simulink model "c00020M_harness"  (R2018a)
settings: Solver=ode3  StartTime=0.0  StopTime=10.0  RelTol=1e-3  EnableMultiTasking=on
undefined symbols (not defined in the file): b, DiscIntNeverNeededParam, J, K, L, PosMinimaW4, R, sigbuilder_block
(part 13 of 41)

== system c00020M_harness/M116/S1 ==
  PhyMeasure : Inport
  SensorOut : Outport
  wires:
  PhyMeasure/1 -> SensorOut/1

== system c00020M_harness/M116/S2 ==
  PhyMeasure : Inport
  SensorOut : Outport
  wires:
  PhyMeasure/1 -> SensorOut/1

== system c00020M_harness/M116/S4 ==
  PhyMeasure : Inport
  SensorOut : Outport
  wires:
  PhyMeasure/1 -> SensorOut/1

== system c00020M_harness/M118/Cyber ==
  note: Sensors
  note: Inputs For Window1
  note: Inputs for Window 2
  note: Inputs for window 3
  note: Inputs for window 4
  note: Users
  note: Users
  note: Sensors
  note: Users
  note: Sensors
  note: Users
  note: Sensors
  note: USERS
      | ---------------------------------
      | 0: None
      | 1: Ventana Arriba
      | 2: Ventana hasta arriba
      | 3: Ventana abajo
      | 4: Ventana hasta abajo
  note: 1: SUBE
      | 0: PARADO
      | -1 BAJA
  note: D = Driver (W1)
      | P1 = Passenger 1 (W2)
      | P2 = Passenger 2 (W3)
      | P3 = Passenger 3 (W4)
      | O = Obstacle
      | C = Control
      | Pri = Prioritizer
      | LD = LockDriver
      | PosW = PositionWindow
      | WL = WindowLogic
      | OW = ObstacleWindow
      | CWXC = ControlWindowXCentralized
      | S = Sensor
      | L = Lock
      | WPos = WindowPosition
      | M = Memory
      | InW = InputWindow
      | WIn = WindowInput
  PosW1 : Inport
  PosW2 : Inport  Port=2
  PosW4 : Inport  Port=3
  DW1 : Inport  Port=4
  DW4 : Inport  Port=5
  P1W2 : Inport  Port=6
  P3W4 : Inport  Port=7
  OW1 : Inport  Port=8
  OW2 : Inport  Port=9
  OW4 : Inport  Port=10
  LD : Inport  Port=11
  Pri4 : Subsystem
  WL : Subsystem
  WL1 : Subsystem
  WL3 : Subsystem
  W1 : Outport
  W2 : Outport  Port=2
  W4 : Outport  Port=3
  wires:
  WL3/1(WindowLogicOutput) -> W4/1
  Pri4/1(User) -> WL3/2(User)
  OW4/1 -> WL3/3(OW)
  PosW4/1 -> WL3/1(WPos)
  P3W4/1 -> Pri4/2(P)
  DW4/1 -> Pri4/1(D)
  WL1/1(WindowLogicOutput) -> W2/1
  OW2/1 -> WL1/3(OW)
  PosW2/1 -> WL1/1(WPos)
  WL/1(WindowLogicOutput) -> W1/1
  OW1/1 -> WL/3(OW)
  PosW1/1 -> WL/1(WPos)
  LD/1 -> WL3/4(L)
  DW1/1 -> WL/2(User)
  P1W2/1 -> WL1/2(User)

== system c00020M_harness/M118/Physical ==
  InW1 : Inport
  InW2 : Inport  Port=2
  InW4 : Inport  Port=3
  W : Subsystem
  W5 : Subsystem
  W7 : Subsystem
  W1 : Outport
  W2 : Outport  Port=2
  W4 : Outport  Port=3
  wires:
  W7/1(WPos) -> W4/1
  W5/1(WPos) -> W2/1
  W/1(WPos) -> W1/1
  InW4/1 -> W7/1(WIn)
  InW2/1 -> W5/1(WIn)
  InW1/1 -> W/1(WIn)

== system c00020M_harness/M118/S1 ==
  PhyMeasure : Inport
  SensorOut : Outport
  wires:
  PhyMeasure/1 -> SensorOut/1

== system c00020M_harness/M118/S2 ==
  PhyMeasure : Inport
  SensorOut : Outport
  wires:
  PhyMeasure/1 -> SensorOut/1

== system c00020M_harness/M118/S4 ==
  PhyMeasure : Inport
  SensorOut : Outport
  wires:
  PhyMeasure/1 -> SensorOut/1

== system c00020M_harness/M119/Cyber ==
  note: Sensors
  note: Inputs For Window1
  note: Inputs for Window 2
  note: Inputs for window 3
  note: Inputs for window 4
  note: Users
  note: Users
  note: Sensors
  note: Users
  note: Sensors
  note: Users
  note: Sensors
  note: USERS
      | ---------------------------------
      | 0: None
      | 1: Ventana Arriba
      | 2: Ventana hasta arriba
      | 3: Ventana abajo
      | 4: Ventana hasta abajo
  note: 1: SUBE
      | 0: PARADO
      | -1 BAJA
  note: D = Driver (W1)
      | P1 = Passenger 1 (W2)
      | P2 = Passenger 2 (W3)
      | P3 = Passenger 3 (W4)
      | O = Obstacle
      | C = Control
      | Pri = Prioritizer
      | LD = LockDriver
      | PosW = PositionWindow
      | WL = WindowLogic
      | OW = ObstacleWindow
      | CWXC = ControlWindowXCentralized
      | S = Sensor
      | L = Lock
      | WPos = WindowPosition
      | M = Memory
      | InW = InputWindow
      | WIn = WindowInput
  PosW1 : Inport
  PosW2 : Inport  Port=2
  PosW4 : Inport  Port=3
  DW1 : Inport  Port=4
  DW4 : Inport  Port=5
  P1W2 : Inport  Port=6
  P3W4 : Inport  Port=7
  OW1 : Inport  Port=8
  OW2 : Inport  Port=9
  OW4 : Inport  Port=10
  LD : Inport  Port=11
  Pri4 : Subsystem
  WL : Subsystem
  WL1 : Subsystem
  WL3 : Subsystem
  W1 : Outport
  W2 : Outport  Port=2
  W4 : Outport  Port=3
  wires:
  WL3/1(WindowLogicOutput) -> W4/1
  Pri4/1(User) -> WL3/2(User)
  OW4/1 -> WL3/3(OW)
  PosW4/1 -> WL3/1(WPos)
  P3W4/1 -> Pri4/2(P)
  DW4/1 -> Pri4/1(D)
  WL1/1(WindowLogicOutput) -> W2/1
  OW2/1 -> WL1/3(OW)
  PosW2/1 -> WL1/1(WPos)
  WL/1(WindowLogicOutput) -> W1/1
  OW1/1 -> WL/3(OW)
  PosW1/1 -> WL/1(WPos)
  LD/1 -> WL3/4(L)
  DW1/1 -> WL/2(User)
  P1W2/1 -> WL1/2(User)

== system c00020M_harness/M119/Physical ==
  InW1 : Inport
  InW2 : Inport  Port=2
  InW4 : Inport  Port=3
  W : Subsystem
  W5 : Subsystem
  W7 : Subsystem
  W1 : Outport
  W2 : Outport  Port=2
  W4 : Outport  Port=3
  wires:
  W7/1(WPos) -> W4/1
  W5/1(WPos) -> W2/1
  W/1(WPos) -> W1/1
  InW4/1 -> W7/1(WIn)
  InW2/1 -> W5/1(WIn)
  InW1/1 -> W/1(WIn)

== system c00020M_harness/M119/S1 ==
  PhyMeasure : Inport
  SensorOut : Outport
  wires:
  PhyMeasure/1 -> SensorOut/1

== system c00020M_harness/M119/S2 ==
  PhyMeasure : Inport
  SensorOut : Outport
  wires:
  PhyMeasure/1 -> SensorOut/1

== system c00020M_harness/M119/S4 ==
  PhyMeasure : Inport
  SensorOut : Outport
  wires:
  PhyMeasure/1 -> SensorOut/1

== system c00020M_harness/M120/Cyber ==
  note: Sensors
  note: Inputs For Window1
  note: Inputs for Window 2
  note: Inputs for window 3
  note: Inputs for window 4
  note: Users
  note: Users
  note: Sensors
  note: Users
  note: Sensors
  note: Users
  note: Sensors
  note: USERS
      | ---------------------------------
      | 0: None
      | 1: Ventana Arriba
      | 2: Ventana hasta arriba
      | 3: Ventana abajo
      | 4: Ventana hasta abajo
  note: 1: SUBE
      | 0: PARADO
      | -1 BAJA
  note: D = Driver (W1)
      | P1 = Passenger 1 (W2)
      | P2 = Passenger 2 (W3)
      | P3 = Passenger 3 (W4)
      | O = Obstacle
      | C = Control
      | Pri = Prioritizer
      | LD = LockDriver
      | PosW = PositionWindow
      | WL = WindowLogic
      | OW = ObstacleWindow
      | CWXC = ControlWindowXCentralized
      | S = Sensor
      | L = Lock
      | WPos = WindowPosition
      | M = Memory
      | InW = InputWindow
      | WIn = WindowInput
  PosW1 : Inport
  PosW2 : Inport  Port=2
  PosW4 : Inport  Port=3
  DW1 : Inport  Port=4
  DW4 : Inport  Port=5
  P1W2 : Inport  Port=6
  P3W4 : Inport  Port=7
  OW1 : Inport  Port=8
  OW2 : Inport  Port=9
  OW4 : Inport  Port=10
  LD : Inport  Port=11
  Pri4 : Subsystem
  WL : Subsystem
  WL1 : Subsystem
  WL3 : Subsystem
  W1 : Outport
  W2 : Outport  Port=2
  W4 : Outport  Port=3
  wires:
  WL3/1(WindowLogicOutput) -> W4/1
  Pri4/1(User) -> WL3/2(User)
  OW4/1 -> WL3/3(OW)
  PosW4/1 -> WL3/1(WPos)
  P3W4/1 -> Pri4/2(P)
  DW4/1 -> Pri4/1(D)
  WL1/1(WindowLogicOutput) -> W2/1
  OW2/1 -> WL1/3(OW)
  PosW2/1 -> WL1/1(WPos)
  WL/1(WindowLogicOutput) -> W1/1
  OW1/1 -> WL/3(OW)
  PosW1/1 -> WL/1(WPos)
  LD/1 -> WL3/4(L)
  DW1/1 -> WL/2(User)
  P1W2/1 -> WL1/2(User)

== system c00020M_harness/M120/Physical ==
  InW1 : Inport
  InW2 : Inport  Port=2
  InW4 : Inport  Port=3
  W : Subsystem
  W5 : Subsystem
  W7 : Subsystem
  W1 : Outport
  W2 : Outport  Port=2
  W4 : Outport  Port=3
  wires:
  W7/1(WPos) -> W4/1
  W5/1(WPos) -> W2/1
  W/1(WPos) -> W1/1
  InW4/1 -> W7/1(WIn)
  InW2/1 -> W5/1(WIn)
  InW1/1 -> W/1(WIn)

== system c00020M_harness/M120/S1 ==
  PhyMeasure : Inport
  SensorOut : Outport
  wires:
  PhyMeasure/1 -> SensorOut/1

== system c00020M_harness/M120/S2 ==
  PhyMeasure : Inport
  SensorOut : Outport
  wires:
  PhyMeasure/1 -> SensorOut/1

== system c00020M_harness/M120/S4 ==
  PhyMeasure : Inport
  SensorOut : Outport
  wires:
  PhyMeasure/1 -> SensorOut/1

== system c00020M_harness/M122/Cyber ==
  note: Sensors
  note: Inputs For Window1
  note: Inputs for Window 2
  note: Inputs for window 3
  note: Inputs for window 4
  note: Users
  note: Users
  note: Sensors
  note: Users
  note: Sensors
  note: Users
  note: Sensors
  note: USERS
      | ---------------------------------
      | 0: None
      | 1: Ventana Arriba
      | 2: Ventana hasta arriba
      | 3: Ventana abajo
      | 4: Ventana hasta abajo
  note: 1: SUBE
      | 0: PARADO
      | -1 BAJA
  note: D = Driver (W1)
      | P1 = Passenger 1 (W2)
      | P2 = Passenger 2 (W3)
      | P3 = Passenger 3 (W4)
      | O = Obstacle
      | C = Control
      | Pri = Prioritizer
      | LD = LockDriver
      | PosW = PositionWindow
      | WL = WindowLogic
      | OW = ObstacleWindow
      | CWXC = ControlWindowXCentralized
      | S = Sensor
      | L = Lock
      | WPos = WindowPosition
      | M = Memory
      | InW = InputWindow
      | WIn = WindowInput
  PosW1 : Inport
  PosW2 : Inport  Port=2
  PosW4 : Inport  Port=3
  DW1 : Inport  Port=4
  DW4 : Inport  Port=5
  P1W2 : Inport  Port=6
  P3W4 : Inport  Port=7
  OW1 : Inport  Port=8
  OW2 : Inport  Port=9
  OW4 : Inport  Port=10
  LD : Inport  Port=11
  Pri4 : Subsystem
  WL : Subsystem
  WL1 : Subsystem
  WL3 : Subsystem
  W1 : Outport
  W2 : Outport  Port=2
  W4 : Outport  Port=3
  wires:
  WL3/1(WindowLogicOutput) -> W4/1
  Pri4/1(User) -> WL3/2(User)
  OW4/1 -> WL3/3(OW)
  PosW4/1 -> WL3/1(WPos)
  P3W4/1 -> Pri4/2(P)
  DW4/1 -> Pri4/1(D)
  WL1/1(WindowLogicOutput) -> W2/1
  OW2/1 -> WL1/3(OW)
  PosW2/1 -> WL1/1(WPos)
  WL/1(WindowLogicOutput) -> W1/1
  OW1/1 -> WL/3(OW)
  PosW1/1 -> WL/1(WPos)
  LD/1 -> WL3/4(L)
  DW1/1 -> WL/2(User)
  P1W2/1 -> WL1/2(User)

== system c00020M_harness/M122/Physical ==
  InW1 : Inport
  InW2 : Inport  Port=2
  InW4 : Inport  Port=3
  W : Subsystem
  W5 : Subsystem
  W7 : Subsystem
  W1 : Outport
  W2 : Outport  Port=2
  W4 : Outport  Port=3
  wires:
  W7/1(WPos) -> W4/1
  W5/1(WPos) -> W2/1
  W/1(WPos) -> W1/1
  InW4/1 -> W7/1(WIn)
  InW2/1 -> W5/1(WIn)
  InW1/1 -> W/1(WIn)

== system c00020M_harness/M122/S1 ==
  PhyMeasure : Inport
  SensorOut : Outport
  wires:
  PhyMeasure/1 -> SensorOut/1

== system c00020M_harness/M122/S2 ==
  PhyMeasure : Inport
  SensorOut : Outport
  wires:
  PhyMeasure/1 -> SensorOut/1

== system c00020M_harness/M122/S4 ==
  PhyMeasure : Inport
  SensorOut : Outport
  wires:
  PhyMeasure/1 -> SensorOut/1

== system c00020M_harness/M123/Cyber ==
  note: Sensors
  note: Inputs For Window1
  note: Inputs for Window 2
  note: Inputs for window 3
  note: Inputs for window 4
  note: Users
  note: Users
  note: Sensors
  note: Users
  note: Sensors
  note: Users
  note: Sensors
  note: USERS
      | ---------------------------------
      | 0: None
      | 1: Ventana Arriba
      | 2: Ventana hasta arriba
      | 3: Ventana abajo
      | 4: Ventana hasta abajo
  note: 1: SUBE
      | 0: PARADO
      | -1 BAJA
  note: D = Driver (W1)
      | P1 = Passenger 1 (W2)
      | P2 = Passenger 2 (W3)
      | P3 = Passenger 3 (W4)
      | O = Obstacle
      | C = Control
      | Pri = Prioritizer
      | LD = LockDriver
      | PosW = PositionWindow
      | WL = WindowLogic
      | OW = ObstacleWindow
      | CWXC = ControlWindowXCentralized
      | S = Sensor
      | L = Lock
      | WPos = WindowPosition
      | M = Memory
      | InW = InputWindow
      | WIn = WindowInput
  PosW1 : Inport
  PosW2 : Inport  Port=2
  PosW4 : Inport  Port=3
  DW1 : Inport  Port=4
  DW4 : Inport  Port=5
  P1W2 : Inport  Port=6
  P3W4 : Inport  Port=7
  OW1 : Inport  Port=8
  OW2 : Inport  Port=9
  OW4 : Inport  Port=10
  LD : Inport  Port=11
  Pri4 : Subsystem
  WL : Subsystem
  WL1 : Subsystem
  WL3 : Subsystem
  W1 : Outport
  W2 : Outport  Port=2
  W4 : Outport  Port=3
  wires:
  WL3/1(WindowLogicOutput) -> W4/1
  Pri4/1(User) -> WL3/2(User)
  OW4/1 -> WL3/3(OW)
  PosW4/1 -> WL3/1(WPos)
  P3W4/1 -> Pri4/2(P)
  DW4/1 -> Pri4/1(D)
  WL1/1(WindowLogicOutput) -> W2/1
  OW2/1 -> WL1/3(OW)
  PosW2/1 -> WL1/1(WPos)
  WL/1(WindowLogicOutput) -> W1/1
  OW1/1 -> WL/3(OW)
  PosW1/1 -> WL/1(WPos)
  LD/1 -> WL3/4(L)
  DW1/1 -> WL/2(User)
  P1W2/1 -> WL1/2(User)

== system c00020M_harness/M123/Physical ==
  InW1 : Inport
  InW2 : Inport  Port=2
  InW4 : Inport  Port=3
  W : Subsystem
  W5 : Subsystem
  W7 : Subsystem
  W1 : Outport
  W2 : Outport  Port=2
  W4 : Outport  Port=3
  wires:
  W7/1(WPos) -> W4/1
  W5/1(WPos) -> W2/1
  W/1(WPos) -> W1/1
  InW4/1 -> W7/1(WIn)
  InW2/1 -> W5/1(WIn)
  InW1/1 -> W/1(WIn)

== system c00020M_harness/M123/S1 ==
  PhyMeasure : Inport
  SensorOut : Outport
  wires:
  PhyMeasure/1 -> SensorOut/1

== system c00020M_harness/M123/S2 ==
  PhyMeasure : Inport
  SensorOut : Outport
  wires:
  PhyMeasure/1 -> SensorOut/1

== system c00020M_harness/M123/S4 ==
  PhyMeasure : Inport
  SensorOut : Outport
  wires:
  PhyMeasure/1 -> SensorOut/1

== system c00020M_harness/M124/Cyber ==
  note: Sensors
  note: Inputs For Window1
  note: Inputs for Window 2
  note: Inputs for window 3
  note: Inputs for window 4
  note: Users
  note: Users
  note: Sensors
  note: Users
  note: Sensors
  note: Users
  note: Sensors
  note: USERS
      | ---------------------------------
      | 0: None
      | 1: Ventana Arriba
      | 2: Ventana hasta arriba
      | 3: Ventana abajo
      | 4: Ventana hasta abajo
  note: 1: SUBE
      | 0: PARADO
      | -1 BAJA
  note: D = Driver (W1)
      | P1 = Passenger 1 (W2)
      | P2 = Passenger 2 (W3)
      | P3 = Passenger 3 (W4)
      | O = Obstacle
      | C = Control
      | Pri = Prioritizer
      | LD = LockDriver
      | PosW = PositionWindow
      | WL = WindowLogic
      | OW = ObstacleWindow
      | CWXC = ControlWindowXCentralized
      | S = Sensor
      | L = Lock
      | WPos = WindowPosition
      | M = Memory
      | InW = InputWindow
      | WIn = WindowInput
  PosW1 : Inport
  PosW2 : Inport  Port=2
  PosW4 : Inport  Port=3
  DW1 : Inport  Port=4
  DW4 : Inport  Port=5
  P1W2 : Inport  Port=6
  P3W4 : Inport  Port=7
  OW1 : Inport  Port=8
  OW2 : Inport  Port=9
  OW4 : Inport  Port=10
  LD : Inport  Port=11
  Pri4 : Subsystem
  WL : Subsystem
  WL1 : Subsystem
  WL3 : Subsystem
  W1 : Outport
  W2 : Outport  Port=2
  W4 : Outport  Port=3
  wires:
  WL3/1(WindowLogicOutput) -> W4/1
  Pri4/1(User) -> WL3/2(User)
  OW4/1 -> WL3/3(OW)
  PosW4/1 -> WL3/1(WPos)
  P3W4/1 -> Pri4/2(P)
  DW4/1 -> Pri4/1(D)
  WL1/1(WindowLogicOutput) -> W2/1
  OW2/1 -> WL1/3(OW)
  PosW2/1 -> WL1/1(WPos)
  WL/1(WindowLogicOutput) -> W1/1
  OW1/1 -> WL/3(OW)
  PosW1/1 -> WL/1(WPos)
  LD/1 -> WL3/4(L)
  DW1/1 -> WL/2(User)
  P1W2/1 -> WL1/2(User)

== system c00020M_harness/M124/Physical ==
  InW1 : Inport
  InW2 : Inport  Port=2
  InW4 : Inport  Port=3
  W : Subsystem
  W5 : Subsystem
  W7 : Subsystem
  W1 : Outport
  W2 : Outport  Port=2
  W4 : Outport  Port=3
  wires:
  W7/1(WPos) -> W4/1
  W5/1(WPos) -> W2/1
  W/1(WPos) -> W1/1
  InW4/1 -> W7/1(WIn)
  InW2/1 -> W5/1(WIn)
  InW1/1 -> W/1(WIn)

== system c00020M_harness/M124/S1 ==
  PhyMeasure : Inport
  SensorOut : Outport
  wires:
  PhyMeasure/1 -> SensorOut/1

== system c00020M_harness/M124/S2 ==
  PhyMeasure : Inport
  SensorOut : Outport
  wires:
  PhyMeasure/1 -> SensorOut/1

== system c00020M_harness/M124/S4 ==
  PhyMeasure : Inport
  SensorOut : Outport
  wires:
  PhyMeasure/1 -> SensorOut/1

== system c00020M_harness/M126/Cyber ==
  note: Sensors
  note: Inputs For Window1
  note: Inputs for Window 2
  note: Inputs for window 3
  note: Inputs for window 4
  note: Users
  note: Users
  note: Sensors
  note: Users
  note: Sensors
  note: Users
  note: Sensors
  note: USERS
      | ---------------------------------
      | 0: None
      | 1: Ventana Arriba
      | 2: Ventana hasta arriba
      | 3: Ventana abajo
      | 4: Ventana hasta abajo
  note: 1: SUBE
      | 0: PARADO
      | -1 BAJA
  note: D = Driver (W1)
      | P1 = Passenger 1 (W2)
      | P2 = Passenger 2 (W3)
      | P3 = Passenger 3 (W4)
      | O = Obstacle
      | C = Control
      | Pri = Prioritizer
      | LD = LockDriver
      | PosW = PositionWindow
      | WL = WindowLogic
      | OW = ObstacleWindow
      | CWXC = ControlWindowXCentralized
      | S = Sensor
      | L = Lock
      | WPos = WindowPosition
      | M = Memory
      | InW = InputWindow
      | WIn = WindowInput
  PosW1 : Inport
  PosW2 : Inport  Port=2
  PosW4 : Inport  Port=3
  DW1 : Inport  Port=4
  DW4 : Inport  Port=5
  P1W2 : Inport  Port=6
  P3W4 : Inport  Port=7
  OW1 : Inport  Port=8
  OW2 : Inport  Port=9
  OW4 : Inport  Port=10
  LD : Inport  Port=11
  Pri4 : Subsystem
  WL : Subsystem
  WL1 : Subsystem
  WL3 : Subsystem
  W1 : Outport
  W2 : Outport  Port=2
  W4 : Outport  Port=3
  wires:
  WL3/1(WindowLogicOutput) -> W4/1
  Pri4/1(User) -> WL3/2(User)
  OW4/1 -> WL3/3(OW)
  PosW4/1 -> WL3/1(WPos)
  P3W4/1 -> Pri4/2(P)
  DW4/1 -> Pri4/1(D)
  WL1/1(WindowLogicOutput) -> W2/1
  OW2/1 -> WL1/3(OW)
  PosW2/1 -> WL1/1(WPos)
  WL/1(WindowLogicOutput) -> W1/1
  OW1/1 -> WL/3(OW)
  PosW1/1 -> WL/1(WPos)
  LD/1 -> WL3/4(L)
  DW1/1 -> WL/2(User)
  P1W2/1 -> WL1/2(User)

== system c00020M_harness/M126/Physical ==
  InW1 : Inport
  InW2 : Inport  Port=2
  InW4 : Inport  Port=3
  W : Subsystem
  W5 : Subsystem
  W7 : Subsystem
  W1 : Outport
  W2 : Outport  Port=2
  W4 : Outport  Port=3
  wires:
  W7/1(WPos) -> W4/1
  W5/1(WPos) -> W2/1
  W/1(WPos) -> W1/1
  InW4/1 -> W7/1(WIn)
  InW2/1 -> W5/1(WIn)
  InW1/1 -> W/1(WIn)

== system c00020M_harness/M126/S1 ==
  PhyMeasure : Inport
  SensorOut : Outport
  wires:
  PhyMeasure/1 -> SensorOut/1

== system c00020M_harness/M126/S2 ==
  PhyMeasure : Inport
  SensorOut : Outport
  wires:
  PhyMeasure/1 -> SensorOut/1

== system c00020M_harness/M126/S4 ==
  PhyMeasure : Inport
  SensorOut : Outport
  wires:
  PhyMeasure/1 -> SensorOut/1

== system c00020M_harness/M127/Cyber ==
  note: Sensors
  note: Inputs For Window1
  note: Inputs for Window 2
  note: Inputs for window 3
  note: Inputs for window 4
  note: Users
  note: Users
  note: Sensors
  note: Users
  note: Sensors
  note: Users
  note: Sensors
  note: USERS
      | ---------------------------------
      | 0: None
      | 1: Ventana Arriba
      | 2: Ventana hasta arriba
      | 3: Ventana abajo
      | 4: Ventana hasta abajo
  note: 1: SUBE
      | 0: PARADO
      | -1 BAJA
  note: D = Driver (W1)
      | P1 = Passenger 1 (W2)
      | P2 = Passenger 2 (W3)
      | P3 = Passenger 3 (W4)
      | O = Obstacle
      | C = Control
      | Pri = Prioritizer
      | LD = LockDriver
      | PosW = PositionWindow
      | WL = WindowLogic
      | OW = ObstacleWindow
      | CWXC = ControlWindowXCentralized
      | S = Sensor
      | L = Lock
      | WPos = WindowPosition
      | M = Memory
      | InW = InputWindow
      | WIn = WindowInput
  PosW1 : Inport
  PosW2 : Inport  Port=2
  PosW4 : Inport  Port=3
  DW1 : Inport  Port=4
  DW4 : Inport  Port=5
  P1W2 : Inport  Port=6
  P3W4 : Inport  Port=7
  OW1 : Inport  Port=8
  OW2 : Inport  Port=9
  OW4 : Inport  Port=10
  LD : Inport  Port=11
  Pri4 : Subsystem
  WL : Subsystem
  WL1 : Subsystem
  WL3 : Subsystem
  W1 : Outport
  W2 : Outport  Port=2
  W4 : Outport  Port=3
  wires:
  WL3/1(WindowLogicOutput) -> W4/1
  Pri4/1(User) -> WL3/2(User)
  OW4/1 -> WL3/3(OW)
  PosW4/1 -> WL3/1(WPos)
  P3W4/1 -> Pri4/2(P)
  DW4/1 -> Pri4/1(D)
  WL1/1(WindowLogicOutput) -> W2/1
  OW2/1 -> WL1/3(OW)
  PosW2/1 -> WL1/1(WPos)
  WL/1(WindowLogicOutput) -> W1/1
  OW1/1 -> WL/3(OW)
  PosW1/1 -> WL/1(WPos)
  LD/1 -> WL3/4(L)
  DW1/1 -> WL/2(User)
  P1W2/1 -> WL1/2(User)

== system c00020M_harness/M127/Physical ==
  InW1 : Inport
  InW2 : Inport  Port=2
  InW4 : Inport  Port=3
  W : Subsystem
  W5 : Subsystem
  W7 : Subsystem
  W1 : Outport
  W2 : Outport  Port=2
  W4 : Outport  Port=3
  wires:
  W7/1(WPos) -> W4/1
  W5/1(WPos) -> W2/1
  W/1(WPos) -> W1/1
  InW4/1 -> W7/1(WIn)
  InW2/1 -> W5/1(WIn)
  InW1/1 -> W/1(WIn)

== system c00020M_harness/M127/S1 ==
  PhyMeasure : Inport
  SensorOut : Outport
  wires:
  PhyMeasure/1 -> SensorOut/1

== system c00020M_harness/M127/S2 ==
  PhyMeasure : Inport
  SensorOut : Outport
  wires:
  PhyMeasure/1 -> SensorOut/1

== system c00020M_harness/M127/S4 ==
  PhyMeasure : Inport
  SensorOut : Outport
  wires:
  PhyMeasure/1 -> SensorOut/1

== system c00020M_harness/M128/Cyber ==
  note: Sensors
  note: Inputs For Window1
  note: Inputs for Window 2
  note: Inputs for window 3
  note: Inputs for window 4
  note: Users
  note: Users
  note: Sensors
  note: Users
  note: Sensors
  note: Users
  note: Sensors
  note: USERS
      | ---------------------------------
      | 0: None
      | 1: Ventana Arriba
      | 2: Ventana hasta arriba
      | 3: Ventana abajo
      | 4: Ventana hasta abajo
  note: 1: SUBE
      | 0: PARADO
      | -1 BAJA
  note: D = Driver (W1)
      | P1 = Passenger 1 (W2)
      | P2 = Passenger 2 (W3)
      | P3 = Passenger 3 (W4)
      | O = Obstacle
      | C = Control
      | Pri = Prioritizer
      | LD = LockDriver
      | PosW = PositionWindow
      | WL = WindowLogic
      | OW = ObstacleWindow
      | CWXC = ControlWindowXCentralized
      | S = Sensor
      | L = Lock
      | WPos = WindowPosition
      | M = Memory
      | InW = InputWindow
      | WIn = WindowInput
  PosW1 : Inport
  PosW2 : Inport  Port=2
  PosW4 : Inport  Port=3
  DW1 : Inport  Port=4
  DW4 : Inport  Port=5
  P1W2 : Inport  Port=6
  P3W4 : Inport  Port=7
  OW1 : Inport  Port=8
  OW2 : Inport  Port=9
  OW4 : Inport  Port=10
  LD : Inport  Port=11
  Pri4 : Subsystem
  WL : Subsystem
  WL1 : Subsystem
  WL3 : Subsystem
  W1 : Outport
  W2 : Outport  Port=2
  W4 : Outport  Port=3
  wires:
  WL3/1(WindowLogicOutput) -> W4/1
  Pri4/1(User) -> WL3/2(User)
  OW4/1 -> WL3/3(OW)
  PosW4/1 -> WL3/1(WPos)
  P3W4/1 -> Pri4/2(P)
  DW4/1 -> Pri4/1(D)
  WL1/1(WindowLogicOutput) -> W2/1
  OW2/1 -> WL1/3(OW)
  PosW2/1 -> WL1/1(WPos)
  WL/1(WindowLogicOutput) -> W1/1
  OW1/1 -> WL/3(OW)
  PosW1/1 -> WL/1(WPos)
  LD/1 -> WL3/4(L)
  DW1/1 -> WL/2(User)
  P1W2/1 -> WL1/2(User)

== system c00020M_harness/M128/Physical ==
  InW1 : Inport
  InW2 : Inport  Port=2
  InW4 : Inport  Port=3
  W : Subsystem
  W5 : Subsystem
  W7 : Subsystem
  W1 : Outport
  W2 : Outport  Port=2
  W4 : Outport  Port=3
  wires:
  W7/1(WPos) -> W4/1
  W5/1(WPos) -> W2/1
  W/1(WPos) -> W1/1
  InW4/1 -> W7/1(WIn)
  InW2/1 -> W5/1(WIn)
  InW1/1 -> W/1(WIn)

== system c00020M_harness/M128/S1 ==
  PhyMeasure : Inport
  SensorOut : Outport
  wires:
  PhyMeasure/1 -> SensorOut/1

== system c00020M_harness/M128/S2 ==
  PhyMeasure : Inport
  SensorOut : Outport
  wires:
  PhyMeasure/1 -> SensorOut/1

== system c00020M_harness/M128/S4 ==
  PhyMeasure : Inport
  SensorOut : Outport
  wires:
  PhyMeasure/1 -> SensorOut/1

== system c00020M_harness/M130/Cyber ==
  note: Sensors
  note: Inputs For Window1
  note: Inputs for Window 2
  note: Inputs for window 3
  note: Inputs for window 4
  note: Users
  note: Users
  note: Sensors
  note: Users
  note: Sensors
  note: Users
  note: Sensors
  note: USERS
      | ---------------------------------
      | 0: None
      | 1: Ventana Arriba
      | 2: Ventana hasta arriba
      | 3: Ventana abajo
      | 4: Ventana hasta abajo
  note: 1: SUBE
      | 0: PARADO
      | -1 BAJA
  note: D = Driver (W1)
      | P1 = Passenger 1 (W2)
      | P2 = Passenger 2 (W3)
      | P3 = Passenger 3 (W4)
      | O = Obstacle
      | C = Control
      | Pri = Prioritizer
      | LD = LockDriver
      | PosW = PositionWindow
      | WL = WindowLogic
      | OW = ObstacleWindow
      | CWXC = ControlWindowXCentralized
      | S = Sensor
      | L = Lock
      | WPos = WindowPosition
      | M = Memory
      | InW = InputWindow
      | WIn = WindowInput
  PosW1 : Inport
  PosW2 : Inport  Port=2
  PosW4 : Inport  Port=3
  DW1 : Inport  Port=4
  DW4 : Inport  Port=5
  P1W2 : Inport  Port=6
  P3W4 : Inport  Port=7
  OW1 : Inport  Port=8
  OW2 : Inport  Port=9
  OW4 : Inport  Port=10
  LD : Inport  Port=11
  Pri4 : Subsystem
  WL : Subsystem
  WL1 : Subsystem
  WL3 : Subsystem
  W1 : Outport
  W2 : Outport  Port=2
  W4 : Outport  Port=3
  wires:
  WL3/1(WindowLogicOutput) -> W4/1
  Pri4/1(User) -> WL3/2(User)
  OW4/1 -> WL3/3(OW)
  PosW4/1 -> WL3/1(WPos)
  P3W4/1 -> Pri4/2(P)
  DW4/1 -> Pri4/1(D)
  WL1/1(WindowLogicOutput) -> W2/1
  OW2/1 -> WL1/3(OW)
  PosW2/1 -> WL1/1(WPos)
  WL/1(WindowLogicOutput) -> W1/1
  OW1/1 -> WL/3(OW)
  PosW1/1 -> WL/1(WPos)
  LD/1 -> WL3/4(L)
  DW1/1 -> WL/2(User)
  P1W2/1 -> WL1/2(User)

== system c00020M_harness/M130/Physical ==
  InW1 : Inport
  InW2 : Inport  Port=2
  InW4 : Inport  Port=3
  W : Subsystem
  W5 : Subsystem
  W7 : Subsystem
  W1 : Outport
  W2 : Outport  Port=2
  W4 : Outport  Port=3
  wires:
  W7/1(WPos) -> W4/1
  W5/1(WPos) -> W2/1
  W/1(WPos) -> W1/1
  InW4/1 -> W7/1(WIn)
  InW2/1 -> W5/1(WIn)
  InW1/1 -> W/1(WIn)

== system c00020M_harness/M130/S1 ==
  PhyMeasure : Inport
  SensorOut : Outport
  wires:
  PhyMeasure/1 -> SensorOut/1

== system c00020M_harness/M130/S2 ==
  PhyMeasure : Inport
  SensorOut : Outport
  wires:
  PhyMeasure/1 -> SensorOut/1

== system c00020M_harness/M130/S4 ==
  PhyMeasure : Inport
  SensorOut : Outport
  wires:
  PhyMeasure/1 -> SensorOut/1

== system c00020M_harness/M131/Cyber ==
  note: Sensors
  note: Inputs For Window1
  note: Inputs for Window 2
  note: Inputs for window 3
  note: Inputs for window 4
  note: Users
  note: Users
  note: Sensors
  note: Users
  note: Sensors
  note: Users
  note: Sensors
  note: USERS
      | ---------------------------------
      | 0: None
      | 1: Ventana Arriba
      | 2: Ventana hasta arriba
      | 3: Ventana abajo
      | 4: Ventana hasta abajo
  note: 1: SUBE
      | 0: PARADO
      | -1 BAJA
  note: D = Driver (W1)
      | P1 = Passenger 1 (W2)
      | P2 = Passenger 2 (W3)
      | P3 = Passenger 3 (W4)
      | O = Obstacle
      | C = Control
      | Pri = Prioritizer
      | LD = LockDriver
      | PosW = PositionWindow
      | WL = WindowLogic
      | OW = ObstacleWindow
      | CWXC = ControlWindowXCentralized
      | S = Sensor
      | L = Lock
      | WPos = WindowPosition
      | M = Memory
      | InW = InputWindow
      | WIn = WindowInput
  PosW1 : Inport
  PosW2 : Inport  Port=2
  PosW4 : Inport  Port=3
  DW1 : Inport  Port=4
  DW4 : Inport  Port=5
  P1W2 : Inport  Port=6
  P3W4 : Inport  Port=7
  OW1 : Inport  Port=8
  OW2 : Inport  Port=9
  OW4 : Inport  Port=10
  LD : Inport  Port=11
  Pri4 : Subsystem
  WL : Subsystem
  WL1 : Subsystem
  WL3 : Subsystem
  W1 : Outport
  W2 : Outport  Port=2
  W4 : Outport  Port=3
  wires:
  WL3/1(WindowLogicOutput) -> W4/1
  Pri4/1(User) -> WL3/2(User)
  OW4/1 -> WL3/3(OW)
  PosW4/1 -> WL3/1(WPos)
  P3W4/1 -> Pri4/2(P)
  DW4/1 -> Pri4/1(D)
  WL1/1(WindowLogicOutput) -> W2/1
  OW2/1 -> WL1/3(OW)
  PosW2/1 -> WL1/1(WPos)
  WL/1(WindowLogicOutput) -> W1/1
  OW1/1 -> WL/3(OW)
  PosW1/1 -> WL/1(WPos)
  LD/1 -> WL3/4(L)
  DW1/1 -> WL/2(User)
  P1W2/1 -> WL1/2(User)

== system c00020M_harness/M131/Physical ==
  InW1 : Inport
  InW2 : Inport  Port=2
  InW4 : Inport  Port=3
  W : Subsystem
  W5 : Subsystem
  W7 : Subsystem
  W1 : Outport
  W2 : Outport  Port=2
  W4 : Outport  Port=3
  wires:
  W7/1(WPos) -> W4/1
  W5/1(WPos) -> W2/1
  W/1(WPos) -> W1/1
  InW4/1 -> W7/1(WIn)
  InW2/1 -> W5/1(WIn)
  InW1/1 -> W/1(WIn)

== system c00020M_harness/M131/S1 ==
  PhyMeasure : Inport
  SensorOut : Outport
  wires:
  PhyMeasure/1 -> SensorOut/1

== system c00020M_harness/M131/S2 ==
  PhyMeasure : Inport
  SensorOut : Outport
  wires:
  PhyMeasure/1 -> SensorOut/1

== system c00020M_harness/M131/S4 ==
  PhyMeasure : Inport
  SensorOut : Outport
  wires:
  PhyMeasure/1 -> SensorOut/1

== system c00020M_harness/M132/Cyber ==
  note: Sensors
  note: Inputs For Window1
  note: Inputs for Window 2
  note: Inputs for window 3
  note: Inputs for window 4
  note: Users
  note: Users
  note: Sensors
  note: Users
  note: Sensors
  note: Users
  note: Sensors
  note: USERS
      | ---------------------------------
      | 0: None
      | 1: Ventana Arriba
      | 2: Ventana hasta arriba
      | 3: Ventana abajo
      | 4: Ventana hasta abajo
  note: 1: SUBE
      | 0: PARADO
      | -1 BAJA
  note: D = Driver (W1)
      | P1 = Passenger 1 (W2)
      | P2 = Passenger 2 (W3)
      | P3 = Passenger 3 (W4)
      | O = Obstacle
      | C = Control
      | Pri = Prioritizer
      | LD = LockDriver
      | PosW = PositionWindow
      | WL = WindowLogic
      | OW = ObstacleWindow
      | CWXC = ControlWindowXCentralized
      | S = Sensor
      | L = Lock
      | WPos = WindowPosition
      | M = Memory
      | InW = InputWindow
      | WIn = WindowInput
  PosW1 : Inport
  PosW2 : Inport  Port=2
  PosW4 : Inport  Port=3
  DW1 : Inport  Port=4
  DW4 : Inport  Port=5
  P1W2 : Inport  Port=6
  P3W4 : Inport  Port=7
  OW1 : Inport  Port=8
  OW2 : Inport  Port=9
  OW4 : Inport  Port=10
  LD : Inport  Port=11
  Pri4 : Subsystem
  WL : Subsystem
  WL1 : Subsystem
  WL3 : Subsystem
  W1 : Outport
  W2 : Outport  Port=2
  W4 : Outport  Port=3
  wires:
  WL3/1(WindowLogicOutput) -> W4/1
  Pri4/1(User) -> WL3/2(User)
  OW4/1 -> WL3/3(OW)
  PosW4/1 -> WL3/1(WPos)
  P3W4/1 -> Pri4/2(P)
  DW4/1 -> Pri4/1(D)
  WL1/1(WindowLogicOutput) -> W2/1
  OW2/1 -> WL1/3(OW)
  PosW2/1 -> WL1/1(WPos)
  WL/1(WindowLogicOutput) -> W1/1
  OW1/1 -> WL/3(OW)
  PosW1/1 -> WL/1(WPos)
  LD/1 -> WL3/4(L)
  DW1/1 -> WL/2(User)
  P1W2/1 -> WL1/2(User)

== system c00020M_harness/M132/Physical ==
  InW1 : Inport
  InW2 : Inport  Port=2
  InW4 : Inport  Port=3
  W : Subsystem
  W5 : Subsystem
  W7 : Subsystem
  W1 : Outport
  W2 : Outport  Port=2
  W4 : Outport  Port=3
  wires:
  W7/1(WPos) -> W4/1
  W5/1(WPos) -> W2/1
  W/1(WPos) -> W1/1
  InW4/1 -> W7/1(WIn)
  InW2/1 -> W5/1(WIn)
  InW1/1 -> W/1(WIn)

== system c00020M_harness/M132/S1 ==
  PhyMeasure : Inport
  SensorOut : Outport
  wires:
  PhyMeasure/1 -> SensorOut/1

== system c00020M_harness/M132/S2 ==
  PhyMeasure : Inport
  SensorOut : Outport
  wires:
  PhyMeasure/1 -> SensorOut/1

== system c00020M_harness/M132/S4 ==
  PhyMeasure : Inport
  SensorOut : Outport
  wires:
  PhyMeasure/1 -> SensorOut/1

== system c00020M_harness/M134/Cyber ==
  note: Sensors
  note: Inputs For Window1
  note: Inputs for Window 2
  note: Inputs for window 3
  note: Inputs for window 4
  note: Users
  note: Users
  note: Sensors
  note: Users
  note: Sensors
  note: Users
  note: Sensors
  note: USERS
      | ---------------------------------
      | 0: None
      | 1: Ventana Arriba
      | 2: Ventana hasta arriba
      | 3: Ventana abajo
      | 4: Ventana hasta abajo
  note: 1: SUBE
      | 0: PARADO
      | -1 BAJA
  note: D = Driver (W1)
      | P1 = Passenger 1 (W2)
      | P2 = Passenger 2 (W3)
      | P3 = Passenger 3 (W4)
      | O = Obstacle
      | C = Control
      | Pri = Prioritizer
      | LD = LockDriver
      | PosW = PositionWindow
      | WL = WindowLogic
      | OW = ObstacleWindow
      | CWXC = ControlWindowXCentralized
      | S = Sensor
      | L = Lock
      | WPos = WindowPosition
      | M = Memory
      | InW = InputWindow
      | WIn = WindowInput
  PosW1 : Inport
  PosW2 : Inport  Port=2
  PosW4 : Inport  Port=3
  DW1 : Inport  Port=4
  DW4 : Inport  Port=5
  P1W2 : Inport  Port=6
  P3W4 : Inport  Port=7
  OW1 : Inport  Port=8
  OW2 : Inport  Port=9
  OW4 : Inport  Port=10
  LD : Inport  Port=11
  Pri4 : Subsystem
  WL : Subsystem
  WL1 : Subsystem
  WL3 : Subsystem
  W1 : Outport
  W2 : Outport  Port=2
  W4 : Outport  Port=3
  wires:
  WL3/1(WindowLogicOutput) -> W4/1
  Pri4/1(User) -> WL3/2(User)
  OW4/1 -> WL3/3(OW)
  PosW4/1 -> WL3/1(WPos)
  P3W4/1 -> Pri4/2(P)
  DW4/1 -> Pri4/1(D)
  WL1/1(WindowLogicOutput) -> W2/1
  OW2/1 -> WL1/3(OW)
  PosW2/1 -> WL1/1(WPos)
  WL/1(WindowLogicOutput) -> W1/1
  OW1/1 -> WL/3(OW)
  PosW1/1 -> WL/1(WPos)
  LD/1 -> WL3/4(L)
  DW1/1 -> WL/2(User)
  P1W2/1 -> WL1/2(User)

== system c00020M_harness/M134/Physical ==
  InW1 : Inport
  InW2 : Inport  Port=2
  InW4 : Inport  Port=3
  W : Subsystem
  W5 : Subsystem
  W7 : Subsystem
  W1 : Outport
  W2 : Outport  Port=2
  W4 : Outport  Port=3
  wires:
  W7/1(WPos) -> W4/1
  W5/1(WPos) -> W2/1
  W/1(WPos) -> W1/1
  InW4/1 -> W7/1(WIn)
  InW2/1 -> W5/1(WIn)
  InW1/1 -> W/1(WIn)

== system c00020M_harness/M134/S1 ==
  PhyMeasure : Inport
  SensorOut : Outport
  wires:
  PhyMeasure/1 -> SensorOut/1

== system c00020M_harness/M134/S2 ==
  PhyMeasure : Inport
  SensorOut : Outport
  wires:
  PhyMeasure/1 -> SensorOut/1

== system c00020M_harness/M134/S4 ==
  PhyMeasure : Inport
  SensorOut : Outport
  wires:
  PhyMeasure/1 -> SensorOut/1

== system c00020M_harness/M135/Cyber ==
  note: Sensors
  note: Inputs For Window1
  note: Inputs for Window 2
  note: Inputs for window 3
  note: Inputs for window 4
  note: Users
  note: Users
  note: Sensors
  note: Users
  note: Sensors
  note: Users
  note: Sensors
  note: USERS
      | ---------------------------------
      | 0: None
      | 1: Ventana Arriba
      | 2: Ventana hasta arriba
      | 3: Ventana abajo
      | 4: Ventana hasta abajo
  note: 1: SUBE
      | 0: PARADO
      | -1 BAJA
  note: D = Driver (W1)
      | P1 = Passenger 1 (W2)
      | P2 = Passenger 2 (W3)
      | P3 = Passenger 3 (W4)
      | O = Obstacle
      | C = Control
      | Pri = Prioritizer
      | LD = LockDriver
      | PosW = PositionWindow
      | WL = WindowLogic
      | OW = ObstacleWindow
      | CWXC = ControlWindowXCentralized
      | S = Sensor
      | L = Lock
      | WPos = WindowPosition
      | M = Memory
      | InW = InputWindow
      | WIn = WindowInput
  PosW1 : Inport
  PosW2 : Inport  Port=2
  PosW4 : Inport  Port=3
  DW1 : Inport  Port=4
  DW4 : Inport  Port=5
  P1W2 : Inport  Port=6
  P3W4 : Inport  Port=7
  OW1 : Inport  Port=8
  OW2 : Inport  Port=9
  OW4 : Inport  Port=10
  LD : Inport  Port=11
  Pri4 : Subsystem
  WL : Subsystem
  WL1 : Subsystem
  WL3 : Subsystem
  W1 : Outport
  W2 : Outport  Port=2
  W4 : Outport  Port=3
  wires:
  WL3/1(WindowLogicOutput) -> W4/1
  Pri4/1(User) -> WL3/2(User)
  OW4/1 -> WL3/3(OW)
  PosW4/1 -> WL3/1(WPos)
  P3W4/1 -> Pri4/2(P)
  DW4/1 -> Pri4/1(D)
  WL1/1(WindowLogicOutput) -> W2/1
  OW2/1 -> WL1/3(OW)
  PosW2/1 -> WL1/1(WPos)
  WL/1(WindowLogicOutput) -> W1/1
  OW1/1 -> WL/3(OW)
  PosW1/1 -> WL/1(WPos)
  LD/1 -> WL3/4(L)
  DW1/1 -> WL/2(User)
  P1W2/1 -> WL1/2(User)

== system c00020M_harness/M135/Physical ==
  InW1 : Inport
  InW2 : Inport  Port=2
  InW4 : Inport  Port=3
  W : Subsystem
  W5 : Subsystem
  W7 : Subsystem
  W1 : Outport
  W2 : Outport  Port=2
  W4 : Outport  Port=3
  wires:
  W7/1(WPos) -> W4/1
  W5/1(WPos) -> W2/1
  W/1(WPos) -> W1/1
  InW4/1 -> W7/1(WIn)
  InW2/1 -> W5/1(WIn)
  InW1/1 -> W/1(WIn)

== system c00020M_harness/M135/S1 ==
  PhyMeasure : Inport
  SensorOut : Outport
  wires:
  PhyMeasure/1 -> SensorOut/1

== system c00020M_harness/M135/S2 ==
  PhyMeasure : Inport
  SensorOut : Outport
  wires:
  PhyMeasure/1 -> SensorOut/1

== system c00020M_harness/M135/S4 ==
  PhyMeasure : Inport
  SensorOut : Outport
  wires:
  PhyMeasure/1 -> SensorOut/1

== system c00020M_harness/M136/Cyber ==
  note: Sensors
  note: Inputs For Window1
  note: Inputs for Window 2
  note: Inputs for window 3
  note: Inputs for window 4
  note: Users
  note: Users
  note: Sensors
  note: Users
  note: Sensors
  note: Users
  note: Sensors
  note: USERS
      | ---------------------------------
      | 0: None
      | 1: Ventana Arriba
      | 2: Ventana hasta arriba
      | 3: Ventana abajo
      | 4: Ventana hasta abajo
  note: 1: SUBE
      | 0: PARADO
      | -1 BAJA
  note: D = Driver (W1)
      | P1 = Passenger 1 (W2)
      | P2 = Passenger 2 (W3)
      | P3 = Passenger 3 (W4)
      | O = Obstacle
      | C = Control
      | Pri = Prioritizer
      | LD = LockDriver
      | PosW = PositionWindow
      | WL = WindowLogic
      | OW = ObstacleWindow
      | CWXC = ControlWindowXCentralized
      | S = Sensor
      | L = Lock
      | WPos = WindowPosition
      | M = Memory
      | InW = InputWindow
      | WIn = WindowInput
  PosW1 : Inport
  PosW2 : Inport  Port=2
  PosW4 : Inport  Port=3
  DW1 : Inport  Port=4
  DW4 : Inport  Port=5
  P1W2 : Inport  Port=6
  P3W4 : Inport  Port=7
  OW1 : Inport  Port=8
  OW2 : Inport  Port=9
  OW4 : Inport  Port=10
  LD : Inport  Port=11
  Pri4 : Subsystem
  WL : Subsystem
  WL1 : Subsystem
  WL3 : Subsystem
  W1 : Outport
  W2 : Outport  Port=2
  W4 : Outport  Port=3
  wires:
  WL3/1(WindowLogicOutput) -> W4/1
  Pri4/1(User) -> WL3/2(User)
  OW4/1 -> WL3/3(OW)
  PosW4/1 -> WL3/1(WPos)
  P3W4/1 -> Pri4/2(P)
  DW4/1 -> Pri4/1(D)
  WL1/1(WindowLogicOutput) -> W2/1
  OW2/1 -> WL1/3(OW)
  PosW2/1 -> WL1/1(WPos)
  WL/1(WindowLogicOutput) -> W1/1
  OW1/1 -> WL/3(OW)
  PosW1/1 -> WL/1(WPos)
  LD/1 -> WL3/4(L)
  DW1/1 -> WL/2(User)
  P1W2/1 -> WL1/2(User)

== system c00020M_harness/M136/Physical ==
  InW1 : Inport
  InW2 : Inport  Port=2
  InW4 : Inport  Port=3
  W : Subsystem
  W5 : Subsystem
  W7 : Subsystem
  W1 : Outport
  W2 : Outport  Port=2
  W4 : Outport  Port=3
  wires:
  W7/1(WPos) -> W4/1
  W5/1(WPos) -> W2/1
  W/1(WPos) -> W1/1
  InW4/1 -> W7/1(WIn)
  InW2/1 -> W5/1(WIn)
  InW1/1 -> W/1(WIn)

== system c00020M_harness/M136/S1 ==
  PhyMeasure : Inport
  SensorOut : Outport
  wires:
  PhyMeasure/1 -> SensorOut/1

== system c00020M_harness/M136/S2 ==
  PhyMeasure : Inport
  SensorOut : Outport
  wires:
  PhyMeasure/1 -> SensorOut/1

== system c00020M_harness/M136/S4 ==
  PhyMeasure : Inport
  SensorOut : Outport
  wires:
  PhyMeasure/1 -> SensorOut/1

== system c00020M_harness/M138/Cyber ==
  note: Sensors
  note: Inputs For Window1
  note: Inputs for Window 2
  note: Inputs for window 3
  note: Inputs for window 4
  note: Users
  note: Users
  note: Sensors
  note: Users
  note: Sensors
  note: Users
  note: Sensors
  note: USERS
      | ---------------------------------
      | 0: None
      | 1: Ventana Arriba
      | 2: Ventana hasta arriba
      | 3: Ventana abajo
      | 4: Ventana hasta abajo
  note: 1: SUBE
      | 0: PARADO
      | -1 BAJA
  note: D = Driver (W1)
      | P1 = Passenger 1 (W2)
      | P2 = Passenger 2 (W3)
      | P3 = Passenger 3 (W4)
      | O = Obstacle
      | C = Control
      | Pri = Prioritizer
      | LD = LockDriver
      | PosW = PositionWindow
      | WL = WindowLogic
      | OW = ObstacleWindow
      | CWXC = ControlWindowXCentralized
      | S = Sensor
      | L = Lock
      | WPos = WindowPosition
      | M = Memory
      | InW = InputWindow
      | WIn = WindowInput
  PosW1 : Inport
  PosW2 : Inport  Port=2
  PosW4 : Inport  Port=3
  DW1 : Inport  Port=4
  DW4 : Inport  Port=5
  P1W2 : Inport  Port=6
  P3W4 : Inport  Port=7
  OW1 : Inport  Port=8
  OW2 : Inport  Port=9
  OW4 : Inport  Port=10
  LD : Inport  Port=11
  Pri4 : Subsystem
  WL : Subsystem
  WL1 : Subsystem
  WL3 : Subsystem
  W1 : Outport
  W2 : Outport  Port=2
  W4 : Outport  Port=3
  wires:
  WL3/1(WindowLogicOutput) -> W4/1
  Pri4/1(User) -> WL3/2(User)
  OW4/1 -> WL3/3(OW)
  PosW4/1 -> WL3/1(WPos)
  P3W4/1 -> Pri4/2(P)
  DW4/1 -> Pri4/1(D)
  WL1/1(WindowLogicOutput) -> W2/1
  OW2/1 -> WL1/3(OW)
  PosW2/1 -> WL1/1(WPos)
  WL/1(WindowLogicOutput) -> W1/1
  OW1/1 -> WL/3(OW)
  PosW1/1 -> WL/1(WPos)
  LD/1 -> WL3/4(L)
  DW1/1 -> WL/2(User)
  P1W2/1 -> WL1/2(User)

== system c00020M_harness/M138/Physical ==
  InW1 : Inport
  InW2 : Inport  Port=2
  InW4 : Inport  Port=3
  W : Subsystem
  W5 : Subsystem
  W7 : Subsystem
  W1 : Outport
  W2 : Outport  Port=2
  W4 : Outport  Port=3
  wires:
  W7/1(WPos) -> W4/1
  W5/1(WPos) -> W2/1
  W/1(WPos) -> W1/1
  InW4/1 -> W7/1(WIn)
  InW2/1 -> W5/1(WIn)
  InW1/1 -> W/1(WIn)

== system c00020M_harness/M138/S1 ==
  PhyMeasure : Inport
  SensorOut : Outport
  wires:
  PhyMeasure/1 -> SensorOut/1

== system c00020M_harness/M138/S2 ==
  PhyMeasure : Inport
  SensorOut : Outport
  wires:
  PhyMeasure/1 -> SensorOut/1

== system c00020M_harness/M138/S4 ==
  PhyMeasure : Inport
  SensorOut : Outport
  wires:
  PhyMeasure/1 -> SensorOut/1

== system c00020M_harness/M139/Cyber ==
  note: Sensors
  note: Inputs For Window1
  note: Inputs for Window 2
  note: Inputs for window 3
  note: Inputs for window 4
  note: Users
  note: Users
  note: Sensors
  note: Users
  note: Sensors
  note: Users
  note: Sensors
  note: USERS
      | ---------------------------------
      | 0: None
      | 1: Ventana Arriba
      | 2: Ventana hasta arriba
      | 3: Ventana abajo
      | 4: Ventana hasta abajo
  note: 1: SUBE
      | 0: PARADO
      | -1 BAJA
  note: D = Driver (W1)
      | P1 = Passenger 1 (W2)
      | P2 = Passenger 2 (W3)
      | P3 = Passenger 3 (W4)
      | O = Obstacle
      | C = Control
      | Pri = Prioritizer
      | LD = LockDriver
      | PosW = PositionWindow
      | WL = WindowLogic
      | OW = ObstacleWindow
      | CWXC = ControlWindowXCentralized
      | S = Sensor
      | L = Lock
      | WPos = WindowPosition
      | M = Memory
      | InW = InputWindow
      | WIn = WindowInput
  PosW1 : Inport
  PosW2 : Inport  Port=2
  PosW4 : Inport  Port=3
  DW1 : Inport  Port=4
  DW4 : Inport  Port=5
  P1W2 : Inport  Port=6
  P3W4 : Inport  Port=7
  OW1 : Inport  Port=8
  OW2 : Inport  Port=9
  OW4 : Inport  Port=10
  LD : Inport  Port=11
  Pri4 : Subsystem
  WL : Subsystem
  WL1 : Subsystem
  WL3 : Subsystem
  W1 : Outport
  W2 : Outport  Port=2
  W4 : Outport  Port=3
  wires:
  WL3/1(WindowLogicOutput) -> W4/1
  Pri4/1(User) -> WL3/2(User)
  OW4/1 -> WL3/3(OW)
  PosW4/1 -> WL3/1(WPos)
  P3W4/1 -> Pri4/2(P)
  DW4/1 -> Pri4/1(D)
  WL1/1(WindowLogicOutput) -> W2/1
  OW2/1 -> WL1/3(OW)
  PosW2/1 -> WL1/1(WPos)
  WL/1(WindowLogicOutput) -> W1/1
  OW1/1 -> WL/3(OW)
  PosW1/1 -> WL/1(WPos)
  LD/1 -> WL3/4(L)
  DW1/1 -> WL/2(User)
  P1W2/1 -> WL1/2(User)

== system c00020M_harness/M139/Physical ==
  InW1 : Inport
  InW2 : Inport  Port=2
  InW4 : Inport  Port=3
  W : Subsystem
  W5 : Subsystem
  W7 : Subsystem
  W1 : Outport
  W2 : Outport  Port=2
  W4 : Outport  Port=3
  wires:
  W7/1(WPos) -> W4/1
  W5/1(WPos) -> W2/1
  W/1(WPos) -> W1/1
  InW4/1 -> W7/1(WIn)
  InW2/1 -> W5/1(WIn)
  InW1/1 -> W/1(WIn)

== system c00020M_harness/M139/S1 ==
  PhyMeasure : Inport
  SensorOut : Outport
  wires:
  PhyMeasure/1 -> SensorOut/1

== system c00020M_harness/M139/S2 ==
  PhyMeasure : Inport
  SensorOut : Outport
  wires:
  PhyMeasure/1 -> SensorOut/1

== system c00020M_harness/M139/S4 ==
  PhyMeasure : Inport
  SensorOut : Outport
  wires:
  PhyMeasure/1 -> SensorOut/1

== system c00020M_harness/M140/Cyber ==
  note: Sensors
  note: Inputs For Window1
  note: Inputs for Window 2
  note: Inputs for window 3
  note: Inputs for window 4
  note: Users
  note: Users
  note: Sensors
  note: Users
  note: Sensors
  note: Users
  note: Sensors
  note: USERS
      | ---------------------------------
      | 0: None
      | 1: Ventana Arriba
      | 2: Ventana hasta arriba
      | 3: Ventana abajo
      | 4: Ventana hasta abajo
  note: 1: SUBE
      | 0: PARADO
      | -1 BAJA
  note: D = Driver (W1)
      | P1 = Passenger 1 (W2)
      | P2 = Passenger 2 (W3)
      | P3 = Passenger 3 (W4)
      | O = Obstacle
      | C = Control
      | Pri = Prioritizer
      | LD = LockDriver
      | PosW = PositionWindow
      | WL = WindowLogic
      | OW = ObstacleWindow
      | CWXC = ControlWindowXCentralized
      | S = Sensor
      | L = Lock
      | WPos = WindowPosition
      | M = Memory
      | InW = InputWindow
      | WIn = WindowInput
  PosW1 : Inport
  PosW2 : Inport  Port=2
  PosW4 : Inport  Port=3
  DW1 : Inport  Port=4
  DW4 : Inport  Port=5
  P1W2 : Inport  Port=6
  P3W4 : Inport  Port=7
  OW1 : Inport  Port=8
  OW2 : Inport  Port=9
  OW4 : Inport  Port=10
  LD : Inport  Port=11
  Pri4 : Subsystem
  WL : Subsystem
  WL1 : Subsystem
  WL3 : Subsystem
  W1 : Outport
  W2 : Outport  Port=2
  W4 : Outport  Port=3
  wires:
  WL3/1(WindowLogicOutput) -> W4/1
  Pri4/1(User) -> WL3/2(User)
  OW4/1 -> WL3/3(OW)
  PosW4/1 -> WL3/1(WPos)
  P3W4/1 -> Pri4/2(P)
  DW4/1 -> Pri4/1(D)
  WL1/1(WindowLogicOutput) -> W2/1
  OW2/1 -> WL1/3(OW)
  PosW2/1 -> WL1/1(WPos)
  WL/1(WindowLogicOutput) -> W1/1
  OW1/1 -> WL/3(OW)
  PosW1/1 -> WL/1(WPos)
  LD/1 -> WL3/4(L)
  DW1/1 -> WL/2(User)
  P1W2/1 -> WL1/2(User)

== system c00020M_harness/M140/Physical ==
  InW1 : Inport
  InW2 : Inport  Port=2
  InW4 : Inport  Port=3
  W : Subsystem
  W5 : Subsystem
  W7 : Subsystem
  W1 : Outport
  W2 : Outport  Port=2
  W4 : Outport  Port=3
  wires:
  W7/1(WPos) -> W4/1
  W5/1(WPos) -> W2/1
  W/1(WPos) -> W1/1
  InW4/1 -> W7/1(WIn)
  InW2/1 -> W5/1(WIn)
  InW1/1 -> W/1(WIn)

== system c00020M_harness/M140/S1 ==
  PhyMeasure : Inport
  SensorOut : Outport
  wires:
  PhyMeasure/1 -> SensorOut/1

== system c00020M_harness/M140/S2 ==
  PhyMeasure : Inport
  SensorOut : Outport
  wires:
  PhyMeasure/1 -> SensorOut/1

== system c00020M_harness/M140/S4 ==
  PhyMeasure : Inport
  SensorOut : Outport
  wires:
  PhyMeasure/1 -> SensorOut/1

== system c00020M_harness/M142/Cyber ==
  note: Sensors
  note: Inputs For Window1
  note: Inputs for Window 2
  note: Inputs for window 3
  note: Inputs for window 4
  note: Users
  note: Users
  note: Sensors
  note: Users
  note: Sensors
  note: Users
  note: Sensors
  note: USERS
      | ---------------------------------
      | 0: None
      | 1: Ventana Arriba
      | 2: Ventana hasta arriba
      | 3: Ventana abajo
      | 4: Ventana hasta abajo
  note: 1: SUBE
      | 0: PARADO
      | -1 BAJA
  note: D = Driver (W1)
      | P1 = Passenger 1 (W2)
      | P2 = Passenger 2 (W3)
      | P3 = Passenger 3 (W4)
      | O = Obstacle
      | C = Control
      | Pri = Prioritizer
      | LD = LockDriver
      | PosW = PositionWindow
      | WL = WindowLogic
      | OW = ObstacleWindow
      | CWXC = ControlWindowXCentralized
      | S = Sensor
      | L = Lock
      | WPos = WindowPosition
      | M = Memory
      | InW = InputWindow
      | WIn = WindowInput
  PosW1 : Inport
  PosW2 : Inport  Port=2
  PosW4 : Inport  Port=3
  DW1 : Inport  Port=4
  DW4 : Inport  Port=5
  P1W2 : Inport  Port=6
  P3W4 : Inport  Port=7
  OW1 : Inport  Port=8
  OW2 : Inport  Port=9
  OW4 : Inport  Port=10
  LD : Inport  Port=11
  Pri4 : Subsystem
  WL : Subsystem
  WL1 : Subsystem
  WL3 : Subsystem
  W1 : Outport
  W2 : Outport  Port=2
  W4 : Outport  Port=3
  wires:
  WL3/1(WindowLogicOutput) -> W4/1
  Pri4/1(User) -> WL3/2(User)
  OW4/1 -> WL3/3(OW)
  PosW4/1 -> WL3/1(WPos)
  P3W4/1 -> Pri4/2(P)
  DW4/1 -> Pri4/1(D)
  WL1/1(WindowLogicOutput) -> W2/1
  OW2/1 -> WL1/3(OW)
  PosW2/1 -> WL1/1(WPos)
  WL/1(WindowLogicOutput) -> W1/1
  OW1/1 -> WL/3(OW)
  PosW1/1 -> WL/1(WPos)
  LD/1 -> WL3/4(L)
  DW1/1 -> WL/2(User)
  P1W2/1 -> WL1/2(User)

== system c00020M_harness/M142/Physical ==
  InW1 : Inport
  InW2 : Inport  Port=2
  InW4 : Inport  Port=3
  W : Subsystem
  W5 : Subsystem
  W7 : Subsystem
  W1 : Outport
  W2 : Outport  Port=2
  W4 : Outport  Port=3
  wires:
  W7/1(WPos) -> W4/1
  W5/1(WPos) -> W2/1
  W/1(WPos) -> W1/1
  InW4/1 -> W7/1(WIn)
  InW2/1 -> W5/1(WIn)
  InW1/1 -> W/1(WIn)

== system c00020M_harness/M142/S1 ==
  PhyMeasure : Inport
  SensorOut : Outport
  wires:
  PhyMeasure/1 -> SensorOut/1

== system c00020M_harness/M142/S2 ==
  PhyMeasure : Inport
  SensorOut : Outport
  wires:
  PhyMeasure/1 -> SensorOut/1

== system c00020M_harness/M142/S4 ==
  PhyMeasure : Inport
  SensorOut : Outport
  wires:
  PhyMeasure/1 -> SensorOut/1

== system c00020M_harness/M143/Cyber ==
  note: Sensors
  note: Inputs For Window1
  note: Inputs for Window 2
  note: Inputs for window 3
  note: Inputs for window 4
  note: Users
  note: Users
  note: Sensors
  note: Users
  note: Sensors
  note: Users
  note: Sensors
  note: USERS
      | ---------------------------------
      | 0: None
      | 1: Ventana Arriba
      | 2: Ventana hasta arriba
      | 3: Ventana abajo
      | 4: Ventana hasta abajo
  note: 1: SUBE
      | 0: PARADO
      | -1 BAJA
  note: D = Driver (W1)
      | P1 = Passenger 1 (W2)
      | P2 = Passenger 2 (W3)
      | P3 = Passenger 3 (W4)
      | O = Obstacle
      | C = Control
      | Pri = Prioritizer
      | LD = LockDriver
      | PosW = PositionWindow
      | WL = WindowLogic
      | OW = ObstacleWindow
      | CWXC = ControlWindowXCentralized
      | S = Sensor
      | L = Lock
      | WPos = WindowPosition
      | M = Memory
      | InW = InputWindow
      | WIn = WindowInput
  PosW1 : Inport
  PosW2 : Inport  Port=2
  PosW4 : Inport  Port=3
  DW1 : Inport  Port=4
  DW4 : Inport  Port=5
  P1W2 : Inport  Port=6
  P3W4 : Inport  Port=7
  OW1 : Inport  Port=8
  OW2 : Inport  Port=9
  OW4 : Inport  Port=10
  LD : Inport  Port=11
  Pri4 : Subsystem
  WL : Subsystem
  WL1 : Subsystem
  WL3 : Subsystem
  W1 : Outport
  W2 : Outport  Port=2
  W4 : Outport  Port=3
  wires:
  WL3/1(WindowLogicOutput) -> W4/1
  Pri4/1(User) -> WL3/2(User)
  OW4/1 -> WL3/3(OW)
  PosW4/1 -> WL3/1(WPos)
  P3W4/1 -> Pri4/2(P)
  DW4/1 -> Pri4/1(D)
  WL1/1(WindowLogicOutput) -> W2/1
  OW2/1 -> WL1/3(OW)
  PosW2/1 -> WL1/1(WPos)
  WL/1(WindowLogicOutput) -> W1/1
  OW1/1 -> WL/3(OW)
  PosW1/1 -> WL/1(WPos)
  LD/1 -> WL3/4(L)
  DW1/1 -> WL/2(User)
  P1W2/1 -> WL1/2(User)

== system c00020M_harness/M143/Physical ==
  InW1 : Inport
  InW2 : Inport  Port=2
  InW4 : Inport  Port=3
  W : Subsystem
  W5 : Subsystem
  W7 : Subsystem
  W1 : Outport
  W2 : Outport  Port=2
  W4 : Outport  Port=3
  wires:
  W7/1(WPos) -> W4/1
  W5/1(WPos) -> W2/1
  W/1(WPos) -> W1/1
  InW4/1 -> W7/1(WIn)
  InW2/1 -> W5/1(WIn)
  InW1/1 -> W/1(WIn)

== system c00020M_harness/M143/S1 ==
  PhyMeasure : Inport
  SensorOut : Outport
  wires:
  PhyMeasure/1 -> SensorOut/1

== system c00020M_harness/M143/S2 ==
  PhyMeasure : Inport
  SensorOut : Outport
  wires:
  PhyMeasure/1 -> SensorOut/1

== system c00020M_harness/M143/S4 ==
  PhyMeasure : Inport
  SensorOut : Outport
  wires:
  PhyMeasure/1 -> SensorOut/1

== system c00020M_harness/M144/Cyber ==
  note: Sensors
  note: Inputs For Window1
  note: Inputs for Window 2
  note: Inputs for window 3
  note: Inputs for window 4
  note: Users
  note: Users
  note: Sensors
  note: Users
  note: Sensors
  note: Users
  note: Sensors
  note: USERS
      | ---------------------------------
      | 0: None
      | 1: Ventana Arriba
      | 2: Ventana hasta arriba
      | 3: Ventana abajo
      | 4: Ventana hasta abajo
  note: 1: SUBE
      | 0: PARADO
      | -1 BAJA
  note: D = Driver (W1)
      | P1 = Passenger 1 (W2)
      | P2 = Passenger 2 (W3)
      | P3 = Passenger 3 (W4)
      | O = Obstacle
      | C = Control
      | Pri = Prioritizer
      | LD = LockDriver
      | PosW = PositionWindow
      | WL = WindowLogic
      | OW = ObstacleWindow
      | CWXC = ControlWindowXCentralized
      | S = Sensor
      | L = Lock
      | WPos = WindowPosition
      | M = Memory
      | InW = InputWindow
      | WIn = WindowInput
  PosW1 : Inport
  PosW2 : Inport  Port=2
  PosW4 : Inport  Port=3
  DW1 : Inport  Port=4
  DW4 : Inport  Port=5
  P1W2 : Inport  Port=6
  P3W4 : Inport  Port=7
  OW1 : Inport  Port=8
  OW2 : Inport  Port=9
  OW4 : Inport  Port=10
  LD : Inport  Port=11
  Pri4 : Subsystem
  WL : Subsystem
  WL1 : Subsystem
  WL3 : Subsystem
  W1 : Outport
  W2 : Outport  Port=2
  W4 : Outport  Port=3
  wires:
  WL3/1(WindowLogicOutput) -> W4/1
  Pri4/1(User) -> WL3/2(User)
  OW4/1 -> WL3/3(OW)
  PosW4/1 -> WL3/1(WPos)
  P3W4/1 -> Pri4/2(P)
  DW4/1 -> Pri4/1(D)
  WL1/1(WindowLogicOutput) -> W2/1
  OW2/1 -> WL1/3(OW)
  PosW2/1 -> WL1/1(WPos)
  WL/1(WindowLogicOutput) -> W1/1
  OW1/1 -> WL/3(OW)
  PosW1/1 -> WL/1(WPos)
  LD/1 -> WL3/4(L)
  DW1/1 -> WL/2(User)
  P1W2/1 -> WL1/2(User)

== system c00020M_harness/M144/Physical ==
  InW1 : Inport
  InW2 : Inport  Port=2
  InW4 : Inport  Port=3
  W : Subsystem
  W5 : Subsystem
  W7 : Subsystem
  W1 : Outport
  W2 : Outport  Port=2
  W4 : Outport  Port=3
  wires:
  W7/1(WPos) -> W4/1
  W5/1(WPos) -> W2/1
  W/1(WPos) -> W1/1
  InW4/1 -> W7/1(WIn)
  InW2/1 -> W5/1(WIn)
  InW1/1 -> W/1(WIn)

== system c00020M_harness/M144/S1 ==
  PhyMeasure : Inport
  SensorOut : Outport
  wires:
  PhyMeasure/1 -> SensorOut/1

== system c00020M_harness/M144/S2 ==
  PhyMeasure : Inport
  SensorOut : Outport
  wires:
  PhyMeasure/1 -> SensorOut/1

== system c00020M_harness/M144/S4 ==
  PhyMeasure : Inport
  SensorOut : Outport
  wires:
  PhyMeasure/1 -> SensorOut/1

== system c00020M_harness/M146/Cyber ==
  note: Sensors
  note: Inputs For Window1
  note: Inputs for Window 2
  note: Inputs for window 3
  note: Inputs for window 4
  note: Users
  note: Users
  note: Sensors
  note: Users
  note: Sensors
  note: Users
  note: Sensors
  note: USERS
      | ---------------------------------
      | 0: None
      | 1: Ventana Arriba
      | 2: Ventana hasta arriba
      | 3: Ventana abajo
      | 4: Ventana hasta abajo
  note: 1: SUBE
      | 0: PARADO
      | -1 BAJA
  note: D = Driver (W1)
      | P1 = Passenger 1 (W2)
      | P2 = Passenger 2 (W3)
      | P3 = Passenger 3 (W4)
      | O = Obstacle
      | C = Control
      | Pri = Prioritizer
      | LD = LockDriver
      | PosW = PositionWindow
      | WL = WindowLogic
      | OW = ObstacleWindow
      | CWXC = ControlWindowXCentralized
      | S = Sensor
      | L = Lock
      | WPos = WindowPosition
      | M = Memory
      | InW = InputWindow
      | WIn = WindowInput
  PosW1 : Inport
  PosW2 : Inport  Port=2
  PosW4 : Inport  Port=3
  DW1 : Inport  Port=4
  DW4 : Inport  Port=5
  P1W2 : Inport  Port=6
  P3W4 : Inport  Port=7
  OW1 : Inport  Port=8
  OW2 : Inport  Port=9
  OW4 : Inport  Port=10
  LD : Inport  Port=11
  Pri4 : Subsystem
  WL : Subsystem
  WL1 : Subsystem
  WL3 : Subsystem
  W1 : Outport
  W2 : Outport  Port=2
  W4 : Outport  Port=3
  wires:
  WL3/1(WindowLogicOutput) -> W4/1
  Pri4/1(User) -> WL3/2(User)
  OW4/1 -> WL3/3(OW)
  PosW4/1 -> WL3/1(WPos)
  P3W4/1 -> Pri4/2(P)
  DW4/1 -> Pri4/1(D)
  WL1/1(WindowLogicOutput) -> W2/1
  OW2/1 -> WL1/3(OW)
  PosW2/1 -> WL1/1(WPos)
  WL/1(WindowLogicOutput) -> W1/1
  OW1/1 -> WL/3(OW)
  PosW1/1 -> WL/1(WPos)
  LD/1 -> WL3/4(L)
  DW1/1 -> WL/2(User)
  P1W2/1 -> WL1/2(User)
